simulink model "Pendulum_Math_Model_Lineal_NoLineal"  (R2020b)
settings: Solver=ode4  StartTime=0.0  StopTime=2.5  FixedStep=0.01  RelTol=1e-3
settings Model: Creator=410  LastModifiedBy=petir

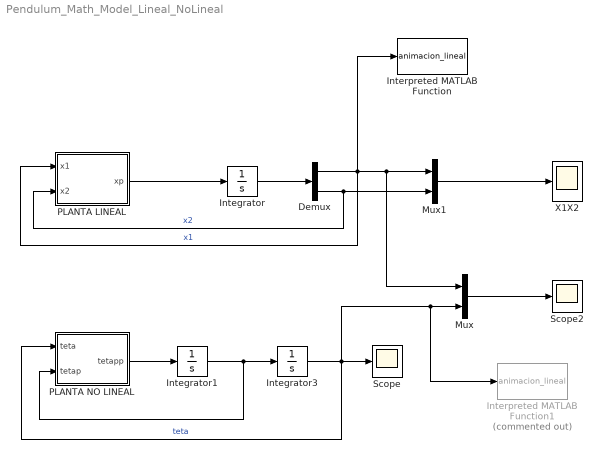
== system Pendulum_Math_Model_Lineal_NoLineal ==
  Demux : Demux  Outputs=2
  Integrator : Integrator  InitialCondition=[pi/4 0]
  Integrator1 : Integrator
  Integrator3 : Integrator  InitialCondition=0.10
  Interpreted MATLAB Function : MATLABFcn  MATLABFcn=animacion_lineal  OutputDimensions=0
  Interpreted MATLAB Function1 : MATLABFcn  Commented=on  MATLABFcn=animacion_lineal  OutputDimensions=0
  Mux : Mux  Inputs=2
  Mux1 : Mux  Inputs=2
  PLANTA LINEAL : MATLAB Function  TreatAsAtomicUnit=on
  PLANTA NO LINEAL : MATLAB Function  TreatAsAtomicUnit=on
  Scope : Scope
  Scope2 : Scope
  X1X2 : Scope
  wires:
  PLANTA LINEAL/1(xp) -> Integrator/1
  Integrator/1 -> Demux/1
  PLANTA NO LINEAL/1(tetapp) -> Integrator1/1
  Demux/1 -> Interpreted MATLAB Function/1, PLANTA LINEAL/1(x1), Mux/1, Mux1/1  "x1"
  Demux/2 -> Mux1/2, PLANTA LINEAL/2(x2)  "x2"
  Integrator1/1 -> Integrator3/1, PLANTA NO LINEAL/2(tetap)
  Integrator3/1 -> Interpreted MATLAB Function1/1, Mux/2, PLANTA NO LINEAL/1(teta), Scope/1  "teta"
  Mux/1 -> Scope2/1
  Mux1/1 -> X1X2/1

== matlab function Pendulum_Math_Model_Lineal_NoLineal/PLANTA LINEAL ==
  data: xp output; x1 input; x2 input
function xp = fcn(x1, x2)
% Parametros
m = 1;
L = 1;
g = 9.81;

% Matrices
A = [0, 1; g/L, 0];
B = [0; 1/(m * L^2)];

% Vector
x = [x1; x2];

% Control
k = [109.81, 16];
u = -k * x;

% Planta
xp = A * x + B * u;

== matlab function Pendulum_Math_Model_Lineal_NoLineal/PLANTA NO LINEAL ==
  data: teta input; tetapp output; tetap input
function tetapp = fcn(teta, tetap)
% PARAMETROS
m = 1;
L = 1;
g = 9.81;

% Control
k = [109.81 16];
x = [teta; tetap];

u = -k*x;
T = u;

% Planta
tetapp = 1 / (m * L^2) * T + g/L * sin(teta);
